simulink model "UAV_Model"  (R2025b)
settings: Solver=ode4  StartTime=0.0  StopTime=50  FixedStep=Step_Size  RelTol=1e-3  EnableMultiTasking=on
values from neighbouring files (symbols this model uses):
  Init_Pos = [ 0.0, 0.0, -100.0 ]    [main_E2.m]
  Init_Rate = [ x_trim(4), x_trim(5), x_trim(6) ]    [main_E2.m]
  Init_Vel = [ x_trim(1), x_trim(2), x_trim(3) ]    [main_E2.m]
  UNIT_GRAV = 9.81    [main_E2.m]
  x_trim = [19.7714170486 1.55747135078e-22 3.01513977975 3.57452064707e-26 1.12807765409e-24 6.034407576e-27 1.79365250696e-25 0.151333968898 -1.40042455829e-45 -2.75841298622e-46 3.7376372575e-41 -5.9107417756e-40]    [model_data.mat]
libraries: UAV_Model_library x24, aerolibconvert2 x3, aerolibtransform2 x2, shared6dofsys x1, sharedutil x1, shared6dof x1
settings Model: Creator=e803534  LastModifiedBy=nhcho
settings SolverCC: AlgebraicLoopSolver=TrustRegion
settings DataIOCC: ReturnWorkspaceOutputs=off
settings OptimizationCC: ReuseModelBlockBuffer=off  LifeSpan=inf
settings DebuggingCC: UnconnectedInputMsg=warning  UnconnectedOutputMsg=warning  UnconnectedLineMsg=warning  SFUnexpectedBacktrackingDiag=warning  SFNoUnconditionalDefaultTransitionDiag=warning  ArithmeticOperatorsInVariantConditions=warning
settings ModelReferenceCC: EnableRefExpFcnMdlSchedulingChecks=on
settings SFSimCC: SimUseLocalCustomCode=off  CustomCodeUndefinedFunction=UseInterfaceOnly
settings RTWCC: RTWUseLocalCustomCode=off  GPUComputeCapability=3.5
settings CodeAppCC: StateflowObjectComments=on
settings GRTTargetCC: TargetLangStandard=C89/C90 (ANSI)
settings ConfigComp: CovMetricSettings=dw  CovSaveCumulativeToWorkspaceVar=on  CovSaveSingleToWorkspaceVar=on  CovExternalEMLEnable=off

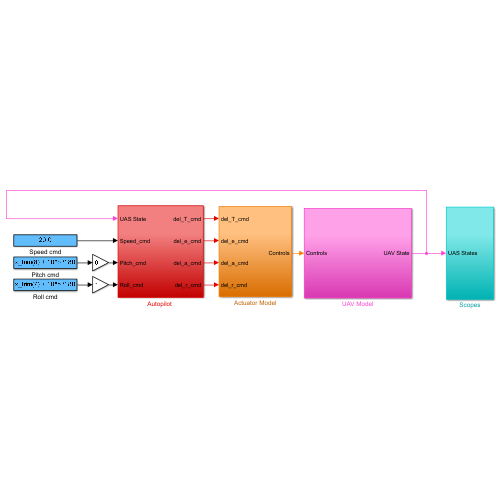
[thumbnail: Simulink's stored preview of the top-level diagram]
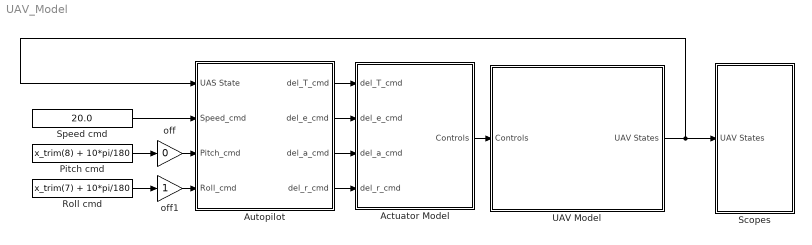
== system UAV_Model ==
  Actuator Model : Subsystem
  "Autopilot " : Subsystem
  Pitch cmd : Constant  Value=x_trim(8) + 10*pi/180
  Roll cmd : Constant  Value=x_trim(7) + 10*pi/180
  Scopes : Subsystem
  Speed cmd : Constant  Value=20.0
  UAV Model : Subsystem
  off : Gain  Gain=0
  off1 : Gain
  wires:
  Actuator Model/1(Controls) -> UAV Model/1(Controls)
  "Autopilot "/1(del_T_cmd) -> Actuator Model/1(del_T_cmd)
  "Autopilot "/2(del_e_cmd) -> Actuator Model/2(del_e_cmd)
  "Autopilot "/3(del_a_cmd) -> Actuator Model/3(del_a_cmd)
  "Autopilot "/4(del_r_cmd) -> Actuator Model/4(del_r_cmd)
  UAV Model/1(UAV States) -> Scopes/1(UAV States), "Autopilot "/1(UAS State)
  Speed cmd/1 -> "Autopilot "/2(Speed_cmd)
  Pitch cmd/1 -> off/1
  Roll cmd/1 -> off1/1
  off/1 -> "Autopilot "/3(Pitch_cmd)
  off1/1 -> "Autopilot "/4(Roll_cmd)

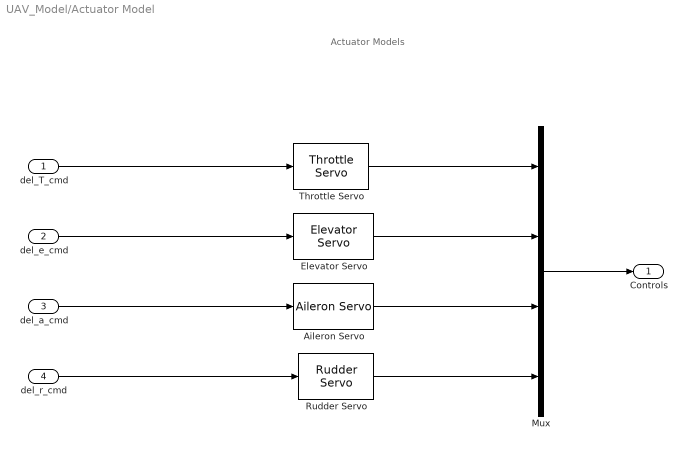
== system UAV_Model/Actuator Model ==
  note: Actuator Models
  del_T_cmd : Inport
  del_e_cmd : Inport  Port=2
  del_a_cmd : Inport  Port=3
  del_r_cmd : Inport  Port=4
  Aileron Servo : UAV_Model_library/Actuator/Aileron Servo  SystemSampleTime=-1  VariantActivationTime=update diagram  EmptyChoice=off  PassThrough=off  PassThroughVariantControl=(default)  EmptyChoiceVariantControl=(default)  AllowFlexibleInterface=on  Latency=0  AutoFrameSizeCalculation=off
  Elevator Servo : UAV_Model_library/Actuator/Elevator Servo  SystemSampleTime=-1  VariantActivationTime=update diagram  EmptyChoice=off  PassThrough=off  PassThroughVariantControl=(default)  EmptyChoiceVariantControl=(default)  AllowFlexibleInterface=on  Latency=0  AutoFrameSizeCalculation=off
  Mux : Mux
  Rudder Servo : UAV_Model_library/Actuator/Rudder Servo  SystemSampleTime=-1  VariantActivationTime=update diagram  EmptyChoice=off  PassThrough=off  PassThroughVariantControl=(default)  EmptyChoiceVariantControl=(default)  AllowFlexibleInterface=on  Latency=0  AutoFrameSizeCalculation=off
  Throttle Servo : UAV_Model_library/Actuator/Throttle Servo  SystemSampleTime=-1  VariantActivationTime=update diagram  EmptyChoice=off  PassThrough=off  PassThroughVariantControl=(default)  EmptyChoiceVariantControl=(default)  AllowFlexibleInterface=on  Latency=0  AutoFrameSizeCalculation=off
  Controls : Outport  VectorParamsAs1DForOutWhenUnconnected=off
  wires:
  del_T_cmd/1 -> Throttle Servo/1
  del_e_cmd/1 -> Elevator Servo/1
  del_a_cmd/1 -> Aileron Servo/1
  del_r_cmd/1 -> Rudder Servo/1
  Elevator Servo/1 -> Mux/2
  Aileron Servo/1 -> Mux/3
  Throttle Servo/1 -> Mux/1
  Rudder Servo/1 -> Mux/4
  Mux/1 -> Controls/1

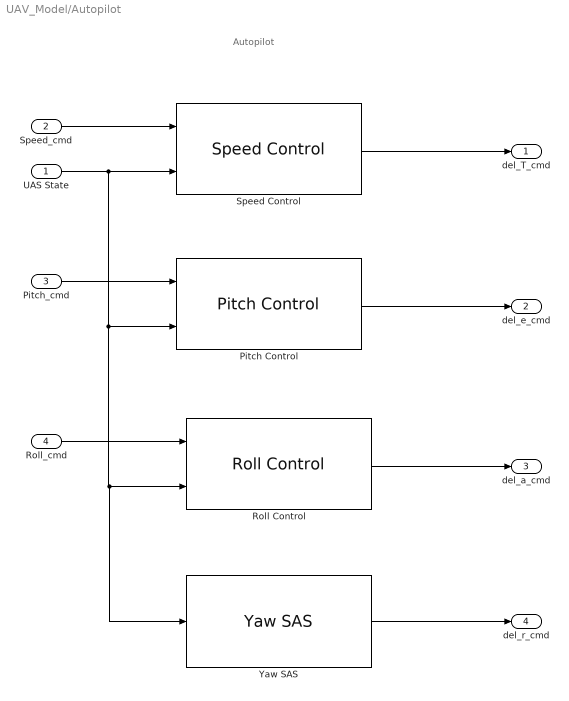
== system UAV_Model/Autopilot  ==
  note: Autopilot
  UAS State : Inport
  Speed_cmd : Inport  Port=2
  Pitch_cmd : Inport  Port=3
  Roll_cmd : Inport  Port=4
  Pitch Control : UAV_Model_library/Autopilot/Pitch Control  SystemSampleTime=-1  VariantActivationTime=update diagram  EmptyChoice=off  PassThrough=off  PassThroughVariantControl=(default)  EmptyChoiceVariantControl=(default)  AllowFlexibleInterface=on  Latency=0  AutoFrameSizeCalculation=off
  Roll Control : UAV_Model_library/Autopilot/Roll Control  SystemSampleTime=-1  VariantActivationTime=update diagram  EmptyChoice=off  PassThrough=off  PassThroughVariantControl=(default)  EmptyChoiceVariantControl=(default)  AllowFlexibleInterface=on  Latency=0  AutoFrameSizeCalculation=off
  Speed Control : UAV_Model_library/Autopilot/Speed Control  SystemSampleTime=-1  VariantActivationTime=update diagram  EmptyChoice=off  PassThrough=off  PassThroughVariantControl=(default)  EmptyChoiceVariantControl=(default)  AllowFlexibleInterface=on  Latency=0  AutoFrameSizeCalculation=off
  Yaw SAS : UAV_Model_library/Autopilot/Yaw SAS  SystemSampleTime=-1  VariantActivationTime=update diagram  EmptyChoice=off  PassThrough=off  PassThroughVariantControl=(default)  EmptyChoiceVariantControl=(default)  AllowFlexibleInterface=on  Latency=0  AutoFrameSizeCalculation=off
  del_T_cmd : Outport  VectorParamsAs1DForOutWhenUnconnected=off
  del_e_cmd : Outport  Port=2  VectorParamsAs1DForOutWhenUnconnected=off
  del_a_cmd : Outport  Port=3  VectorParamsAs1DForOutWhenUnconnected=off
  del_r_cmd : Outport  Port=4  VectorParamsAs1DForOutWhenUnconnected=off
  wires:
  Speed_cmd/1 -> Speed Control/1
  UAS State/1 -> Yaw SAS/1, Roll Control/2, Pitch Control/2, Speed Control/2
  Speed Control/1 -> del_T_cmd/1
  Pitch_cmd/1 -> Pitch Control/1
  Pitch Control/1 -> del_e_cmd/1
  Roll_cmd/1 -> Roll Control/1
  Roll Control/1 -> del_a_cmd/1
  Yaw SAS/1 -> del_r_cmd/1

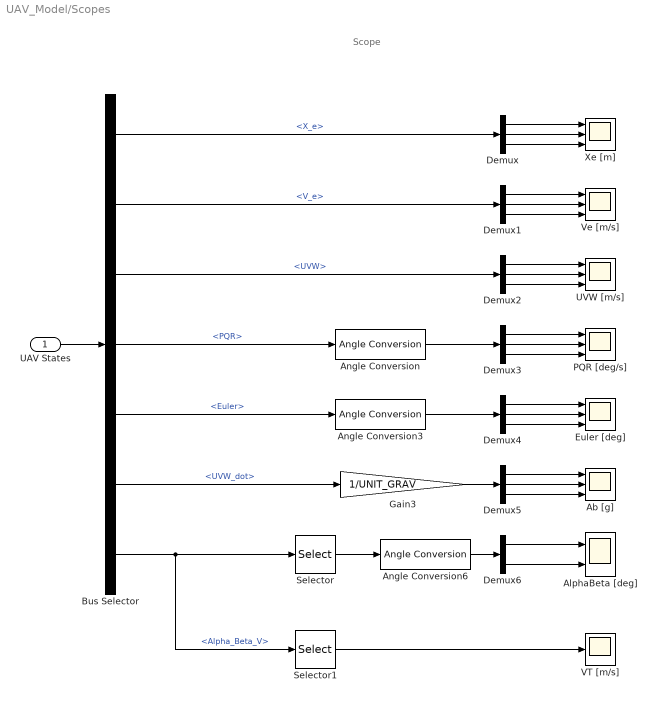
== system UAV_Model/Scopes ==
  note: Scope
  UAV States : Inport
  Ab [g] : Scope  NumInputPorts=3
      settings: ActiveDisplayYMinimum=-0.01356  ActiveDisplayYMaximum=0.06372  DataLoggingSaveFormat=Array
  AlphaBeta [deg] : Scope  NumInputPorts=2
      settings: ActiveDisplayYMinimum=6.34181  ActiveDisplayYMaximum=8.97058  DataLoggingVariableName=Xe15  DataLoggingSaveFormat=Array
  Angle Conversion : aerolibconvert2/Angle Conversion  IU=rad  OU=deg
  Angle Conversion3 : aerolibconvert2/Angle Conversion  IU=rad  OU=deg
  Angle Conversion6 : aerolibconvert2/Angle Conversion  IU=rad  OU=deg
  Bus Selector : BusSelector  OutputSignals=X_e,V_e,UVW,PQR,Euler,UVW_dot,Alpha_Beta_V
  Demux{,1..5} (6 alike) : Demux  Outputs=3
  Demux6 : Demux  Outputs=2
  Euler [deg] : Scope  NumInputPorts=3
      settings: ActiveDisplayYMinimum=-1.24407  ActiveDisplayYMaximum=11.19661  DataLoggingVariableName=Xe12  DataLoggingSaveFormat=Array
  Gain3 : Gain  Gain=1/UNIT_GRAV
  PQR [deg/s] : Scope  NumInputPorts=3
      settings: ActiveDisplayYMinimum=-3.42408  ActiveDisplayYMaximum=27.43519  DataLoggingVariableName=Xe9  DataLoggingSaveFormat=Array
  Selector : Selector  InputPortWidth=3  IndexOptions=Index vector (dialog)  Indices=[1 2]  OutputSizes=1
  Selector1 : Selector  InputPortWidth=3  IndexOptions=Index vector (dialog)  Indices=[3]  OutputSizes=1
  UVW [m/s] : Scope  NumInputPorts=3
      settings: ActiveDisplayYMinimum=19.75177  ActiveDisplayYMaximum=19.94824  DataLoggingVariableName=Xe6  DataLoggingSaveFormat=Array
  VT [m/s] : Scope
      settings: ActiveDisplayYMinimum=19.98078  ActiveDisplayYMaximum=20.17291  DataLoggingVariableName=Xe17  DataLoggingSaveFormat=Array
  Ve [m/s] : Scope  NumInputPorts=3
      settings: ActiveDisplayYMinimum=-24.87948  ActiveDisplayYMaximum=25.03389  DataLoggingVariableName=Xe3  DataLoggingSaveFormat=Array
  Xe [m] : Scope  NumInputPorts=3
      settings: ActiveDisplayYMinimum=-148.42096  ActiveDisplayYMaximum=336.60093  DataLoggingVariableName=Xe  DataLoggingSaveFormat=Array
  wires:
  UAV States/1 -> Bus Selector/1
  Bus Selector/1 -> Demux/1  "<X_e>"
  Bus Selector/2 -> Demux1/1  "<V_e>"
  Bus Selector/3 -> Demux2/1  "<UVW>"
  Bus Selector/4 -> Angle Conversion/1  "<PQR>"
  Bus Selector/5 -> Angle Conversion3/1  "<Euler>"
  Bus Selector/6 -> Gain3/1  "<UVW_dot>"
  Angle Conversion3/1 -> Demux4/1
  Angle Conversion/1 -> Demux3/1
  Selector1/1 -> VT [m/s]/1
  Gain3/1 -> Demux5/1
  Demux/1 -> Xe [m]/1
  Demux/2 -> Xe [m]/2
  Demux/3 -> Xe [m]/3
  Demux1/1 -> Ve [m/s]/1
  Demux1/2 -> Ve [m/s]/2
  Demux1/3 -> Ve [m/s]/3
  Demux2/1 -> UVW [m/s]/1
  Demux2/2 -> UVW [m/s]/2
  Demux2/3 -> UVW [m/s]/3
  Demux3/1 -> PQR [deg/s]/1
  Demux3/2 -> PQR [deg/s]/2
  Demux3/3 -> PQR [deg/s]/3
  Demux4/1 -> Euler [deg]/1
  Demux4/2 -> Euler [deg]/2
  Demux4/3 -> Euler [deg]/3
  Demux5/1 -> Ab [g]/1
  Demux5/2 -> Ab [g]/2
  Demux5/3 -> Ab [g]/3
  Demux6/2 -> AlphaBeta [deg]/2
  Demux6/1 -> AlphaBeta [deg]/1
  Angle Conversion6/1 -> Demux6/1
  Bus Selector/7 -> Selector1/1, Selector/1  "<Alpha_Beta_V>"
  Selector/1 -> Angle Conversion6/1

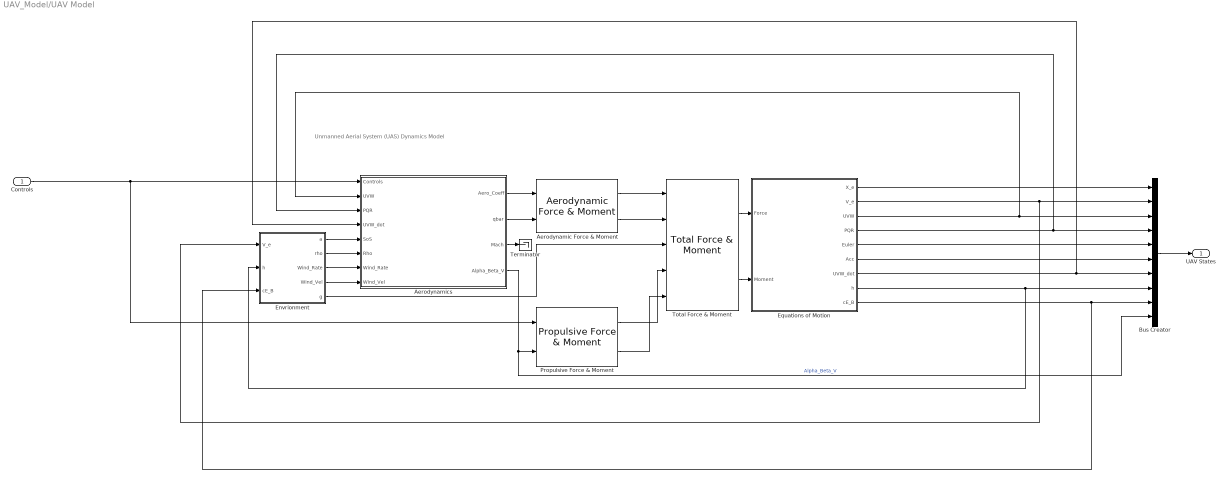
== system UAV_Model/UAV Model ==
  note: Unmanned Aerial System (UAS) Dynamics Model
  Controls : Inport
  Aerodynamic Force & Moment : UAV_Model_library/External Forces/Aerodynamics/Aerodynamic Force & Moment  SystemSampleTime=-1  VariantActivationTime=update diagram  EmptyChoice=off  PassThrough=off  PassThroughVariantControl=(default)  EmptyChoiceVariantControl=(default)  AllowFlexibleInterface=on  Latency=0  AutoFrameSizeCalculation=off
  Aerodynamics : Subsystem
  Bus Creator : BusCreator  Inputs=10
  Envrionment : Subsystem
  Equations of Motion : Subsystem
  Propulsive Force & Moment : UAV_Model_library/External Forces/Propulsive/Propulsive Force & Moment  SystemSampleTime=-1  VariantActivationTime=update diagram  EmptyChoice=off  PassThrough=off  PassThroughVariantControl=(default)  EmptyChoiceVariantControl=(default)  AllowFlexibleInterface=on  Latency=0  AutoFrameSizeCalculation=off
  Terminator : Terminator
  Total Force & Moment : UAV_Model_library/External Forces/Total Force & Moment  SystemSampleTime=-1  VariantActivationTime=update diagram  EmptyChoice=off  PassThrough=off  PassThroughVariantControl=(default)  EmptyChoiceVariantControl=(default)  AllowFlexibleInterface=on  Latency=0  AutoFrameSizeCalculation=off
  UAV States : Outport  VectorParamsAs1DForOutWhenUnconnected=off
  wires:
  Controls/1 -> Propulsive Force & Moment/1, Aerodynamics/1(Controls)
  Bus Creator/1 -> UAV States/1
  Aerodynamic Force & Moment/1 -> Total Force & Moment/1
  Aerodynamic Force & Moment/2 -> Total Force & Moment/2
  Aerodynamics/1(Aero_Coeff) -> Aerodynamic Force & Moment/1
  Aerodynamics/2(qbar) -> Aerodynamic Force & Moment/2
  Aerodynamics/4(Alpha_Beta_V) -> Propulsive Force & Moment/2, Bus Creator/10  "Alpha_Beta_V"
  Envrionment/1(a) -> Aerodynamics/5(SoS)
  Envrionment/2(rho) -> Aerodynamics/6(Rho)
  Envrionment/3(Wind_Rate) -> Aerodynamics/7(Wind_Rate)
  Envrionment/4(Wind_Vel) -> Aerodynamics/8(Wind_Vel)
  Envrionment/5(g) -> Total Force & Moment/3
  Propulsive Force & Moment/1 -> Total Force & Moment/4
  Propulsive Force & Moment/2 -> Total Force & Moment/5
  Total Force & Moment/1 -> Equations of Motion/1(Force)
  Total Force & Moment/2 -> Equations of Motion/2(Moment)
  Equations of Motion/8(h) -> Envrionment/2(h), Bus Creator/8
  Equations of Motion/7(UVW_dot) -> Aerodynamics/4("UVW_dot "), Bus Creator/7
  Equations of Motion/9(cE_B) -> Envrionment/3(cE_B), Bus Creator/9
  Equations of Motion/6(Acc) -> Bus Creator/6
  Equations of Motion/5(Euler) -> Bus Creator/5
  Equations of Motion/4(PQR) -> Aerodynamics/3(PQR), Bus Creator/4
  Equations of Motion/3(UVW) -> Aerodynamics/2(UVW), Bus Creator/3
  Equations of Motion/2(V_e) -> Envrionment/1(V_e), Bus Creator/2
  Equations of Motion/1(X_e) -> Bus Creator/1
  Aerodynamics/3(Mach) -> Terminator/1

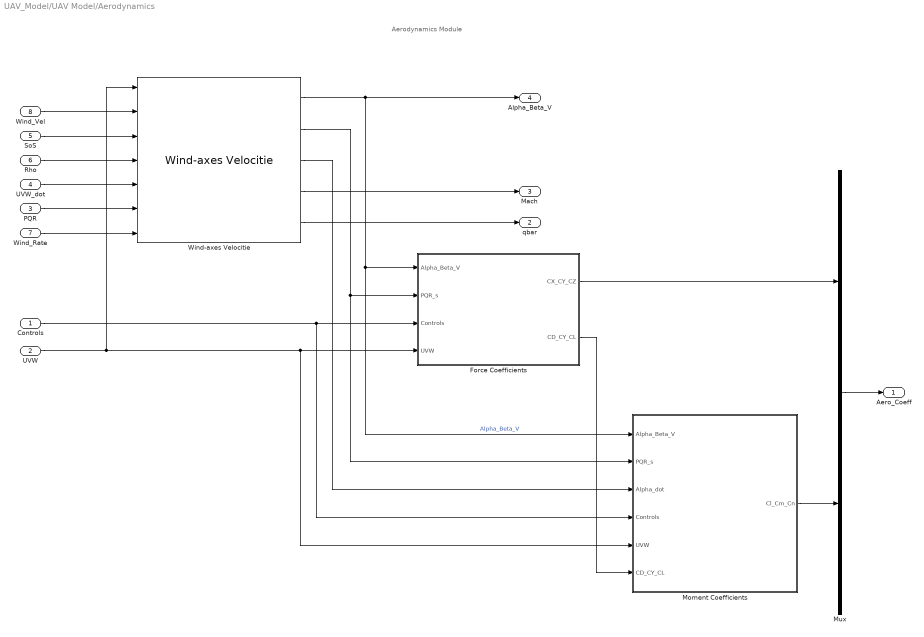
== system UAV_Model/UAV Model/Aerodynamics ==
  note: Aerodynamics Module
  Controls : Inport
  UVW : Inport  Port=2
  PQR : Inport  Port=3
  "UVW_dot " : Inport  Port=4
  SoS : Inport  Port=5
  Rho : Inport  Port=6
  Wind_Rate : Inport  Port=7
  Wind_Vel : Inport  Port=8
  "\tForce Coefficients" : Subsystem
  Moment Coefficients : Subsystem
  Mux : Mux  Inputs=2
  Wind-axes Velocitie : UAV_Model_library/External Forces/Aerodynamics/Wind-axes Velocitie  SystemSampleTime=-1  VariantActivationTime=update diagram  EmptyChoice=off  PassThrough=off  PassThroughVariantControl=(default)  EmptyChoiceVariantControl=(default)  AllowFlexibleInterface=on  Latency=0  AutoFrameSizeCalculation=off
  Aero_Coeff : Outport  VectorParamsAs1DForOutWhenUnconnected=off
  qbar : Outport  Port=2  VectorParamsAs1DForOutWhenUnconnected=off
  Mach : Outport  Port=3  VectorParamsAs1DForOutWhenUnconnected=off
  Alpha_Beta_V : Outport  Port=4  VectorParamsAs1DForOutWhenUnconnected=off
  wires:
  Wind-axes Velocitie/1 -> Alpha_Beta_V/1, Moment Coefficients/1(Alpha_Beta_V), "\tForce Coefficients"/1(Alpha_Beta_V)  "Alpha_Beta_V"
  Wind-axes Velocitie/2 -> Moment Coefficients/2(PQR_s), "\tForce Coefficients"/2(PQR_s)
  Wind-axes Velocitie/3 -> Moment Coefficients/3(Alpha_dot)
  Controls/1 -> "\tForce Coefficients"/3(Controls), Moment Coefficients/4(Controls)
  UVW/1 -> Wind-axes Velocitie/1, Moment Coefficients/5(UVW), "\tForce Coefficients"/4(UVW)
  "\tForce Coefficients"/2("CD_CY_CL ") -> Moment Coefficients/6(CD_CY_CL)
  "\tForce Coefficients"/1(CX_CY_CZ) -> Mux/1
  Moment Coefficients/1(Cl_Cm_Cn) -> Mux/2
  Mux/1 -> Aero_Coeff/1
  Wind-axes Velocitie/4 -> Mach/1
  Wind-axes Velocitie/5 -> qbar/1
  Wind_Vel/1 -> Wind-axes Velocitie/2
  SoS/1 -> Wind-axes Velocitie/3
  Rho/1 -> Wind-axes Velocitie/4
  "UVW_dot "/1 -> Wind-axes Velocitie/5
  PQR/1 -> Wind-axes Velocitie/6
  Wind_Rate/1 -> Wind-axes Velocitie/7

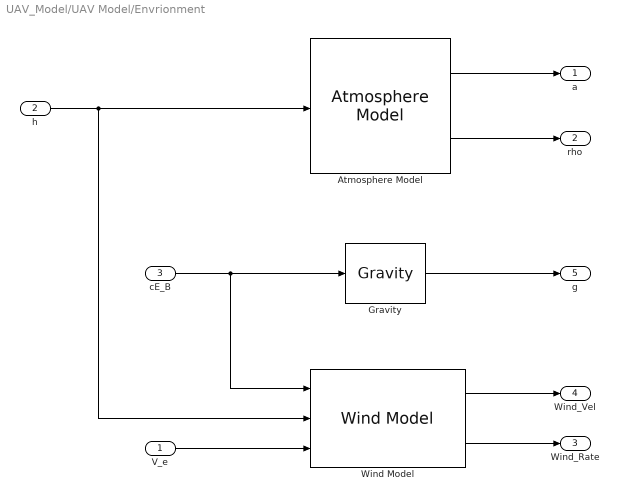
== system UAV_Model/UAV Model/Envrionment ==
  V_e : Inport
  h : Inport  Port=2
  cE_B : Inport  Port=3
  Atmosphere Model : UAV_Model_library/Envrionment/Atmosphere Model  SystemSampleTime=-1  VariantActivationTime=update diagram  EmptyChoice=off  PassThrough=off  PassThroughVariantControl=(default)  EmptyChoiceVariantControl=(default)  AllowFlexibleInterface=on  Latency=0  AutoFrameSizeCalculation=off
  Gravity : UAV_Model_library/Envrionment/Gravity  SystemSampleTime=-1  VariantActivationTime=update diagram  EmptyChoice=off  PassThrough=off  PassThroughVariantControl=(default)  EmptyChoiceVariantControl=(default)  AllowFlexibleInterface=on  Latency=0  AutoFrameSizeCalculation=off
  Wind Model : UAV_Model_library/Envrionment/Wind Model  SystemSampleTime=-1  VariantActivationTime=update diagram  EmptyChoice=off  PassThrough=off  PassThroughVariantControl=(default)  EmptyChoiceVariantControl=(default)  AllowFlexibleInterface=on  Latency=0  AutoFrameSizeCalculation=off
  a : Outport  VectorParamsAs1DForOutWhenUnconnected=off
  rho : Outport  Port=2  VectorParamsAs1DForOutWhenUnconnected=off
  Wind_Rate : Outport  Port=3  VectorParamsAs1DForOutWhenUnconnected=off
  Wind_Vel : Outport  Port=4  VectorParamsAs1DForOutWhenUnconnected=off
  g : Outport  Port=5  VectorParamsAs1DForOutWhenUnconnected=off
  wires:
  h/1 -> Wind Model/2, Atmosphere Model/1
  Atmosphere Model/1 -> a/1
  Atmosphere Model/2 -> rho/1
  cE_B/1 -> Wind Model/1, Gravity/1
  Gravity/1 -> g/1
  V_e/1 -> Wind Model/3
  Wind Model/1 -> Wind_Vel/1
  Wind Model/2 -> Wind_Rate/1

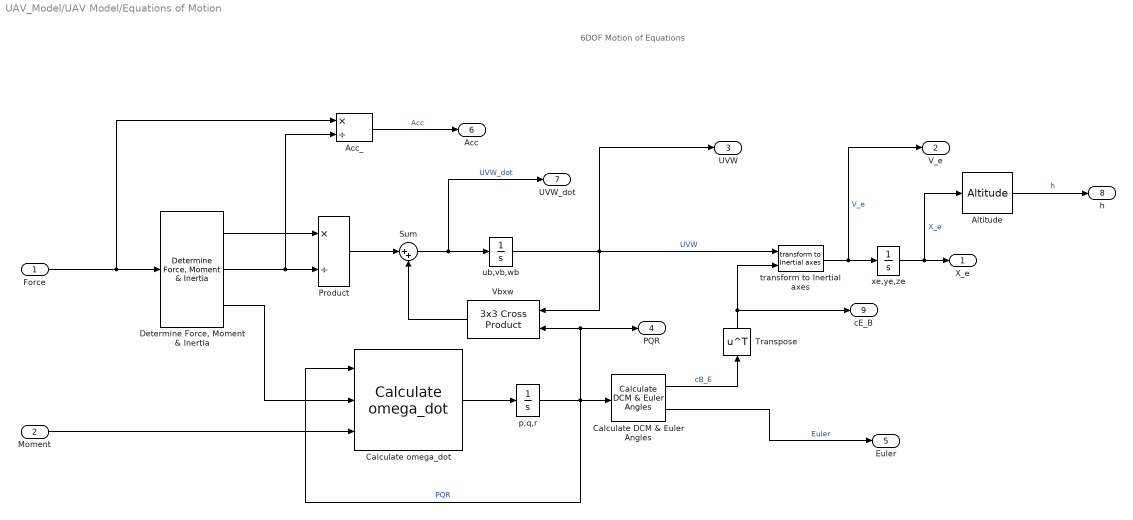
== system UAV_Model/UAV Model/Equations of Motion ==
  note: 6DOF Motion of Equations
  Force : Inport  PortDimensions=3
  Moment : Inport  Port=2  PortDimensions=3
  Acc_ : Product  Inputs=*/  RndMeth=Zero
  Altitude : UAV_Model_library/Equations of Motion/Altitude  SystemSampleTime=-1  VariantActivationTime=update diagram  EmptyChoice=off  PassThrough=off  PassThroughVariantControl=(default)  EmptyChoiceVariantControl=(default)  AllowFlexibleInterface=on  Latency=0  AutoFrameSizeCalculation=off
  Calculate DCM & Euler Angles : UAV_Model_library/Equations of Motion/Calculate DCM & Euler Angles  SystemSampleTime=-1  VariantActivationTime=update diagram  EmptyChoice=off  PassThrough=off  PassThroughVariantControl=(default)  EmptyChoiceVariantControl=(default)  AllowFlexibleInterface=on  Latency=0  AutoFrameSizeCalculation=off
  Calculate omega_dot : shared6dofsys/Calculate omega_dot  aMode=aMode
  "Determine Force, Moment & Inertia" : UAV_Model_library/Equations of Motion/Determine Force, Moment & Inertia  SystemSampleTime=-1  VariantActivationTime=update diagram  EmptyChoice=off  PassThrough=off  PassThroughVariantControl=(default)  EmptyChoiceVariantControl=(default)  AllowFlexibleInterface=on  Latency=0  AutoFrameSizeCalculation=off
  Product : Product  Inputs=*/  SaturateOnIntegerOverflow=on  OutDataTypeStr=Inherit: Same as first input
  Sum : Sum  Inputs=|++  SaturateOnIntegerOverflow=on
  Transpose : Math  Operator=transpose  SignedPower=on
  Vbxw : sharedutil/3x3 Cross Product  aMode=aMode
  "p,q,r " : Integrator  InitialCondition=Init_Rate
  "transform to Inertial axes " : shared6dof/6DOF (Euler Angles)/transform to Inertial axes   SystemSampleTime=-1  VariantActivationTime=update diagram  EmptyChoice=off  PassThrough=off  PassThroughVariantControl=(default)  EmptyChoiceVariantControl=(default)  AllowFlexibleInterface=on  Latency=0  AutoFrameSizeCalculation=off
  ub,vb,wb : Integrator  InitialCondition=Init_Vel
  xe,ye,ze : Integrator  InitialCondition=Init_Pos
  X_e : Outport  VectorParamsAs1DForOutWhenUnconnected=off
  V_e : Outport  Port=2  VectorParamsAs1DForOutWhenUnconnected=off
  UVW : Outport  Port=3  VectorParamsAs1DForOutWhenUnconnected=off
  PQR : Outport  Port=4  VectorParamsAs1DForOutWhenUnconnected=off
  Euler : Outport  Port=5  VectorParamsAs1DForOutWhenUnconnected=off
  Acc : Outport  Port=6  VectorParamsAs1DForOutWhenUnconnected=off
  UVW_dot : Outport  Port=7  VectorParamsAs1DForOutWhenUnconnected=off
  h : Outport  Port=8  VectorParamsAs1DForOutWhenUnconnected=off
  cE_B : Outport  Port=9  VectorParamsAs1DForOutWhenUnconnected=off
  wires:
  Altitude/1 -> h/1  "h"
  Acc_/1 -> Acc/1  "Acc"
  Force/1 -> Acc_/1, "Determine Force, Moment & Inertia"/1
  Sum/1 -> UVW_dot/1, ub,vb,wb/1  "UVW_dot"
  ub,vb,wb/1 -> Vbxw/1, UVW/1, "transform to Inertial axes "/1  "UVW"
  Calculate DCM & Euler Angles/1 -> Transpose/1  "cB_E"
  Calculate DCM & Euler Angles/2 -> Euler/1  "Euler"
  xe,ye,ze/1 -> Altitude/1, X_e/1  "X_e"
  "transform to Inertial axes "/1 -> xe,ye,ze/1, V_e/1  "V_e"
  Moment/1 -> Calculate omega_dot/3
  "Determine Force, Moment & Inertia"/2 -> Product/2, Acc_/2
  Product/1 -> Sum/1
  "Determine Force, Moment & Inertia"/1 -> Product/1
  Vbxw/1 -> Sum/2
  "Determine Force, Moment & Inertia"/3 -> Calculate omega_dot/2
  Calculate omega_dot/1 -> "p,q,r "/1
  "p,q,r "/1 -> PQR/1, Vbxw/2, Calculate omega_dot/1, Calculate DCM & Euler Angles/1  "PQR"
  Transpose/1 -> cE_B/1, "transform to Inertial axes "/2

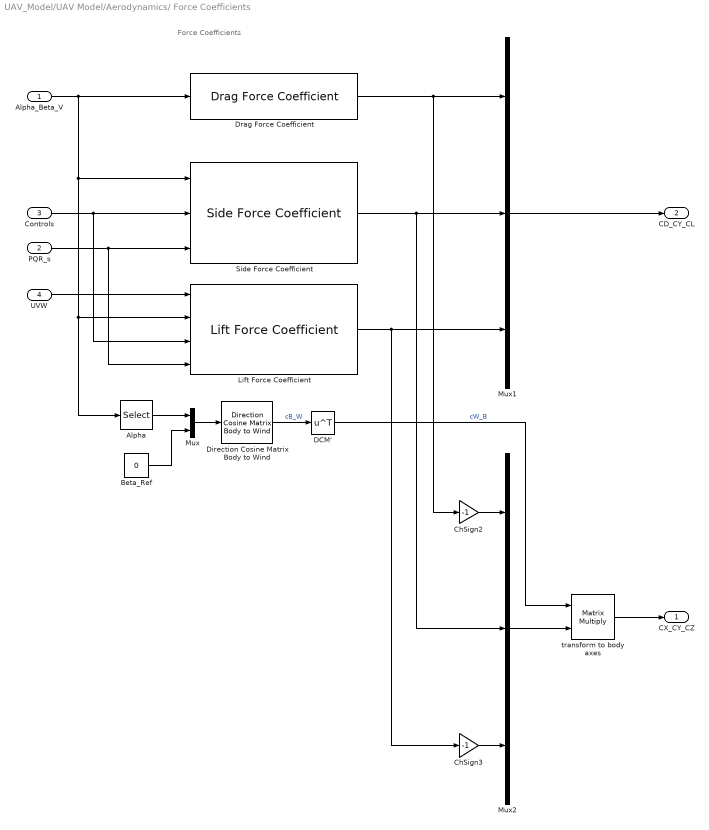
== system UAV_Model/UAV Model/Aerodynamics/	Force Coefficients ==
  note: Force Coefficients
  Alpha_Beta_V : Inport
  PQR_s : Inport  Port=2
  Controls : Inport  Port=3
  UVW : Inport  Port=4
  Alpha : Selector  InputPortWidth=3  IndexOptions=Index vector (dialog)  Indices=[1]  OutputSizes=1
  Beta_Ref : Constant  Value=0
  ChSign2 : Gain  Gain=-1  SaturateOnIntegerOverflow=on  OutDataTypeStr=Inherit: Same as input  ParamDataTypeStr=Inherit: Same as input
  ChSign3 : Gain  Gain=-1  SaturateOnIntegerOverflow=on  OutDataTypeStr=Inherit: Same as input  ParamDataTypeStr=Inherit: Same as input
  DCM' : Math  Operator=transpose  SignedPower=on
  Direction Cosine Matrix Body to Wind : aerolibtransform2/Direction Cosine Matrix Body to Wind
  Drag Force Coefficient : UAV_Model_library/External Forces/Aerodynamics/Aerodynamics coefficients/Drag Force Coefficient  SystemSampleTime=-1  VariantActivationTime=update diagram  EmptyChoice=off  PassThrough=off  PassThroughVariantControl=(default)  EmptyChoiceVariantControl=(default)  AllowFlexibleInterface=on  Latency=0  AutoFrameSizeCalculation=off
  "Lift Force Coefficient  " : UAV_Model_library/External Forces/Aerodynamics/Aerodynamics coefficients/Lift Force Coefficient    SystemSampleTime=-1  VariantActivationTime=update diagram  EmptyChoice=off  PassThrough=off  PassThroughVariantControl=(default)  EmptyChoiceVariantControl=(default)  AllowFlexibleInterface=on  Latency=0  AutoFrameSizeCalculation=off
  Mux : Mux  Inputs=2
  Mux1 : Mux  Inputs=3
  Mux2 : Mux  Inputs=3
  "Side Force Coefficient " : UAV_Model_library/External Forces/Aerodynamics/Aerodynamics coefficients/Side Force Coefficient   SystemSampleTime=-1  VariantActivationTime=update diagram  EmptyChoice=off  PassThrough=off  PassThroughVariantControl=(default)  EmptyChoiceVariantControl=(default)  AllowFlexibleInterface=on  Latency=0  AutoFrameSizeCalculation=off
  transform to body axes : Product  Inputs=**  Multiplication=Matrix(*)  InputSameDT=on  SaturateOnIntegerOverflow=on  OutDataTypeStr=Inherit: Same as first input
  CX_CY_CZ : Outport  VectorParamsAs1DForOutWhenUnconnected=off
  "CD_CY_CL " : Outport  Port=2  VectorParamsAs1DForOutWhenUnconnected=off
  wires:
  Controls/1 -> "Lift Force Coefficient  "/3, "Side Force Coefficient "/2
  PQR_s/1 -> "Lift Force Coefficient  "/4, "Side Force Coefficient "/3
  UVW/1 -> "Lift Force Coefficient  "/1
  Drag Force Coefficient/1 -> ChSign2/1, Mux1/1
  "Side Force Coefficient "/1 -> Mux2/2, Mux1/2
  Mux1/1 -> "CD_CY_CL "/1
  Direction Cosine Matrix Body to Wind/1 -> DCM'/1  "cB_W"
  "Lift Force Coefficient  "/1 -> Mux1/3, ChSign3/1
  ChSign2/1 -> Mux2/1
  ChSign3/1 -> Mux2/3
  DCM'/1 -> transform to body axes/1  "cW_B"
  Mux2/1 -> transform to body axes/2
  transform to body axes/1 -> CX_CY_CZ/1
  Alpha_Beta_V/1 -> Drag Force Coefficient/1, "Side Force Coefficient "/1, "Lift Force Coefficient  "/2, Alpha/1
  Alpha/1 -> Mux/1
  Mux/1 -> Direction Cosine Matrix Body to Wind/1
  Beta_Ref/1 -> Mux/2

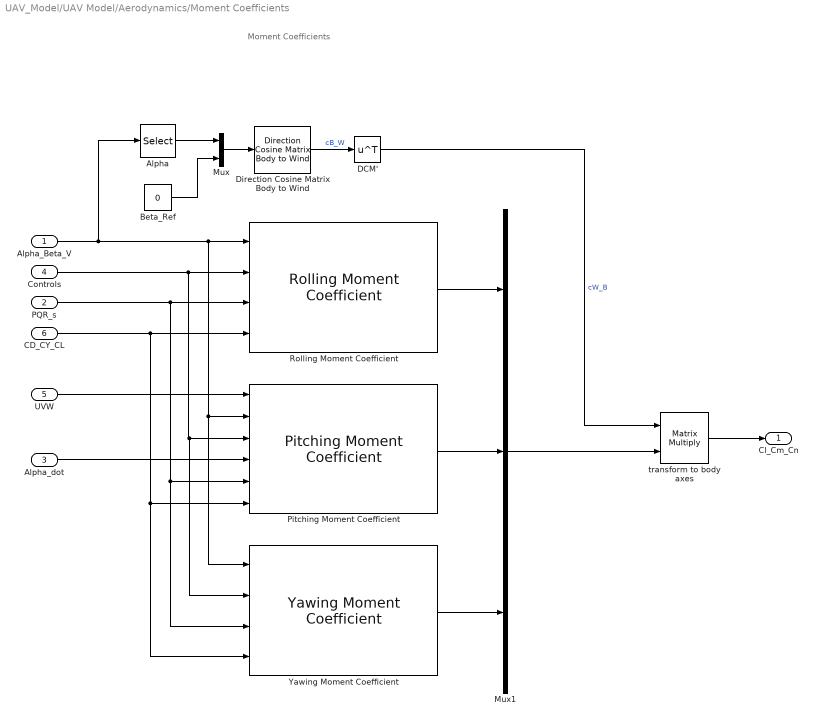
== system UAV_Model/UAV Model/Aerodynamics/Moment Coefficients ==
  note: Moment Coefficients
  Alpha_Beta_V : Inport
  PQR_s : Inport  Port=2
  Alpha_dot : Inport  Port=3
  Controls : Inport  Port=4
  UVW : Inport  Port=5
  CD_CY_CL : Inport  Port=6
  Alpha : Selector  InputPortWidth=3  IndexOptions=Index vector (dialog)  Indices=[1]  OutputSizes=1
  Beta_Ref : Constant  Value=0
  DCM' : Math  Operator=transpose  SignedPower=on
  Direction Cosine Matrix Body to Wind : aerolibtransform2/Direction Cosine Matrix Body to Wind
  Mux : Mux  Inputs=2
  Mux1 : Mux  Inputs=3
  Pitching Moment Coefficient : UAV_Model_library/External Forces/Aerodynamics/Aerodynamics coefficients/Pitching Moment Coefficient  SystemSampleTime=-1  VariantActivationTime=update diagram  EmptyChoice=off  PassThrough=off  PassThroughVariantControl=(default)  EmptyChoiceVariantControl=(default)  AllowFlexibleInterface=on  Latency=0  AutoFrameSizeCalculation=off
  Rolling Moment Coefficient : UAV_Model_library/External Forces/Aerodynamics/Aerodynamics coefficients/Rolling Moment Coefficient  SystemSampleTime=-1  VariantActivationTime=update diagram  EmptyChoice=off  PassThrough=off  PassThroughVariantControl=(default)  EmptyChoiceVariantControl=(default)  AllowFlexibleInterface=on  Latency=0  AutoFrameSizeCalculation=off
  Yawing Moment Coefficient : UAV_Model_library/External Forces/Aerodynamics/Aerodynamics coefficients/Yawing Moment Coefficient  SystemSampleTime=-1  VariantActivationTime=update diagram  EmptyChoice=off  PassThrough=off  PassThroughVariantControl=(default)  EmptyChoiceVariantControl=(default)  AllowFlexibleInterface=on  Latency=0  AutoFrameSizeCalculation=off
  transform to body axes : Product  Inputs=**  Multiplication=Matrix(*)  InputSameDT=on  SaturateOnIntegerOverflow=on  OutDataTypeStr=Inherit: Same as first input
  Cl_Cm_Cn : Outport  VectorParamsAs1DForOutWhenUnconnected=off
  wires:
  Rolling Moment Coefficient/1 -> Mux1/1
  Pitching Moment Coefficient/1 -> Mux1/2
  Mux1/1 -> transform to body axes/2
  Alpha_Beta_V/1 -> Alpha/1, Rolling Moment Coefficient/1, Yawing Moment Coefficient/1, Pitching Moment Coefficient/2
  Controls/1 -> Rolling Moment Coefficient/2, Yawing Moment Coefficient/2, Pitching Moment Coefficient/3
  PQR_s/1 -> Rolling Moment Coefficient/3, Yawing Moment Coefficient/3, Pitching Moment Coefficient/5
  CD_CY_CL/1 -> Rolling Moment Coefficient/4, Yawing Moment Coefficient/4, Pitching Moment Coefficient/6
  UVW/1 -> Pitching Moment Coefficient/1
  Yawing Moment Coefficient/1 -> Mux1/3
  Alpha_dot/1 -> Pitching Moment Coefficient/4
  Direction Cosine Matrix Body to Wind/1 -> DCM'/1  "cB_W"
  Alpha/1 -> Mux/1
  Mux/1 -> Direction Cosine Matrix Body to Wind/1
  Beta_Ref/1 -> Mux/2
  transform to body axes/1 -> Cl_Cm_Cn/1
  DCM'/1 -> transform to body axes/1  "cW_B"
